simulink model "CAVE_MachE_Simulink_250904_Test"  (R2024a)
settings: configuration reference "ConfigSetDesktopFixedStep" (kept outside this file)
PreLoadFcn:
  | VSS_BICYCLE=Simulink.Variant('Dual=0');
  | VSS_DUAL=Simulink.Variant('Dual=1');
  | Dual=1;
  | load('DriveCycle2.mat')
PostLoadFcn:
  | if any(exist('dsrtsu_mdlpostloadfcn', 'file') ~= 0), dsrtsu_mdlpostloadfcn('Execute', bdroot); end
InitFcn:
  | , if any(exist('rtifpga_mdlclblib', 'file') ~= 0), rtifpga_mdlclblib('Init', bdroot); end,
  | , if any(exist('dsmpb_private', 'file') ~= 0), dsmpb_private('dsmpb_mdlclblib', 'Init', bdroot); end,
  | load('DriveCycle2.mat')
model workspace (MAT data in the model file):
  Gas = 0.383333333333
values from neighbouring files (symbols this model uses):
  CoastDown =     [Run_Simulink.mat]
  limitedMCT =     [Run_Simulink.mat]
  MCT =     [Run_Simulink.mat]
  pMCT =     [Run_Simulink.mat]
  RealSimPara =     [Run_Simulink.mat]
  Ref_speed = [13 13.007895099 13.015778396 13.023649891 13.031509584 13.039357475 13.047193564 13.055017851 13.062830336 13.070631019 13.0784199 13.086196979 ... (2669 elements, 2669x1)]    [Ref_speed_and_time.mat]
  Ref_time = [0 0.01 0.02 0.03 0.04 0.05 0.06 0.07 0.08 0.09 0.1 0.11 ... (2669 elements, 2669x1)]    [Ref_speed_and_time.mat]
  US06 =     [Run_Simulink.mat]
undefined symbols (not defined in the file or in its folder): AccelCmd, ActTqLF_Nm_, ActTqLR_Nm_, ActTqRF_Nm_, ActTqRR_Nm_, BattChargeLimitMaxPwr, BattChargeLimitSocBpts, BattChargeLimitTbl, BattChrgCapcty, BattDischargeLimitSocBpts, BattDischargeLimitTbl, BattDischargeMaxPwr, BattNumCellsParallel, BattNumCellsSeries, BattOpenVoltCapBpts, BattOpenVoltTbl, BattResistSocBpts, BattResistTbl, BattResistTempBpts, BrakeMaxPrs, BrakeMaxTrq, ChassisDistCg2FrontAxle, ChassisDistCg2RearAxle, ChassisVehMass, CltchCmd, DecelCmd, DiffRatio, DiscIntNeverNeededParam, EnvGravCnst, EnvPrs, EnvTemp, FuelSpecificGrav, GearCmd, h, InitStates, lgSw, MtrEffSpdBpts, MtrEffTbl, MtrEffTrqBpts, MtrPwrMax, MtrTrqMax, SteeringCmd, SupvsryCtrlRegenBrkCutOffTbl, SupvsryCtrlRegenSpdBpts, TestScnrioCycleNum, VEH
libraries: VSIGenLib x65, simulink x54, etargetslib x38, dsmpblib x24, vehdynlibtire x12, autolibshared x10, vehdynlibsuspension x7, vehdynlibtirecommon x7, autolibutils x5, CarMaker4SL x4, VsrLibWheel x4, autolibpowerinfoutils x3
(part 9 of 16)

== system CAVE_MachE_Simulink_250904_Test/Vehicle Under Test1/Vehicle/Vehicle Dynamics/Vehicle 7DOF/Longitudinal Wheels 4DOF/Tire2Veh ==
  Wheel : Inport
  Bus Selector7 : BusSelector  OutputSignals=Omega,Fx,Re,z,zdot,Kappa,Alpha
  Dead Zone2 : DeadZone  LowerValue=-5  UpperValue=5  ZeroCross=off
  Demux : Demux  Outputs=[2,2]
  Re : Terminator
  Unary Minus1 : UnaryMinus
  Unary Minus2 : UnaryMinus
  zdot : Terminator
  FwF : Outport  VectorParamsAs1DForOutWhenUnconnected=off
  FwR : Outport  Port=2  VectorParamsAs1DForOutWhenUnconnected=off
  z : Outport  Port=3  VectorParamsAs1DForOutWhenUnconnected=off
  Omega : Outport  Port=4  VectorParamsAs1DForOutWhenUnconnected=off
  Kappa : Outport  Port=5  VectorParamsAs1DForOutWhenUnconnected=off
  Alpha : Outport  Port=6  VectorParamsAs1DForOutWhenUnconnected=off
  wires:
  Bus Selector7/7 -> Alpha/1  "<Alpha>"
  Bus Selector7/3 -> Re/1  "<Re>"
  Unary Minus2/1 -> zdot/1  "zdot"
  Bus Selector7/6 -> Kappa/1  "<Kappa>"
  Demux/2 -> FwR/1
  Unary Minus1/1 -> z/1  "z"
  Bus Selector7/4 -> Unary Minus1/1  "<z>"
  Bus Selector7/5 -> Unary Minus2/1  "<zdot>"
  Bus Selector7/1 -> Omega/1  "<Omega>"
  Wheel/1 -> Bus Selector7/1
  Demux/1 -> FwF/1
  Dead Zone2/1 -> Demux/1  "Fx"
  Bus Selector7/2 -> Dead Zone2/1  "<Fx>"

== system CAVE_MachE_Simulink_250904_Test/Vehicle Under Test1/Vehicle/Vehicle Dynamics/Vehicle 7DOF/Longitudinal Wheels 4DOF/Tires ==
  AxlTrq : Inport
  BrkPrs : Inport  Port=2
  Vx : Inport  Port=3
  Vy : Inport  Port=4
  r : Inport  Port=5
  Camber : Inport  Port=6
  TirePrs : Inport  Port=7
  Fz : Inport  Port=8
  lam_mu : Inport  Port=9
  Gnd : Inport  Port=10
  4-by-1 Gnd : Subsystem
  4-by-1 Gnd1 : Subsystem
  4-by-1 Gnd2 : Subsystem
  4-by-1 Gnd3 : Subsystem
  Bus Creator : BusCreator  Inputs=12
  Subsystem : Subsystem
  Terminator1 : Terminator
  Terminator2 : Terminator
  Terminator3 : Terminator
  Wheel : Outport  VectorParamsAs1DForOutWhenUnconnected=off
  wires:
  Gnd/1 -> Subsystem/7(Gnd)
  lam_mu/1 -> Subsystem/6(lam_mu)
  Fz/1 -> Subsystem/5(Fz)
  TirePrs/1 -> Subsystem/4(TirePrs)
  Vx/1 -> Subsystem/3(Vx)
  BrkPrs/1 -> Subsystem/2(BrkPrs)
  AxlTrq/1 -> Subsystem/1(AxlTrq)
  4-by-1 Gnd3/1(Gnd) -> Bus Creator/12  "Alpha"
  Subsystem/8(Kappa) -> Bus Creator/11  "Kappa"
  4-by-1 Gnd2/1(Gnd) -> Bus Creator/7  "Mz"
  4-by-1 Gnd1/1(Gnd) -> Bus Creator/5  "Mx"
  4-by-1 Gnd/1(Gnd) -> Bus Creator/3  "Fy"
  Subsystem/4(My) -> Bus Creator/6  "My"
  Subsystem/3(FzOut) -> Bus Creator/4  "Fz"
  Subsystem/5(Re) -> Bus Creator/8  "Re"
  Subsystem/1(Omega) -> Bus Creator/1  "Omega"
  Subsystem/2(Fx) -> Bus Creator/2  "Fx"
  Subsystem/6(z) -> Bus Creator/9  "z"
  Subsystem/7(zdot) -> Bus Creator/10  "zdot"
  Bus Creator/1 -> Wheel/1
  r/1 -> Terminator3/1
  Camber/1 -> Terminator2/1
  Vy/1 -> Terminator1/1

== system CAVE_MachE_Simulink_250904_Test/Vehicle Under Test1/Vehicle/Vehicle Dynamics/Vehicle 7DOF/Longitudinal Wheels 4DOF/Veh2Tire ==
  AxlTrq : Inport
  BrkPrs : Inport  Port=2
  r : Inport  Port=3
  VehVel : Inport  Port=4
  WhlAng : Inport  Port=5
  Reshape3 : Reshape
  Reshape4 : Reshape
  Unary Minus : UnaryMinus
  Wheel to Body Transform : Subsystem
  T : Outport  VectorParamsAs1DForOutWhenUnconnected=off
  P : Outport  Port=2  VectorParamsAs1DForOutWhenUnconnected=off
  xdotAxle : Outport  Port=3  VectorParamsAs1DForOutWhenUnconnected=off
  ydotAxle : Outport  Port=4  VectorParamsAs1DForOutWhenUnconnected=off
  psidot : Outport  Port=5  VectorParamsAs1DForOutWhenUnconnected=off
  zdotAxle : Outport  Port=6  VectorParamsAs1DForOutWhenUnconnected=off
  wires:
  Reshape3/1 -> P/1
  Unary Minus/1 -> psidot/1
  Wheel to Body Transform/3(zdotWheel) -> zdotAxle/1  "Vz"
  WhlAng/1 -> Wheel to Body Transform/2(WhlAng)
  VehVel/1 -> Wheel to Body Transform/1(VelVeh)
  Reshape4/1 -> T/1
  r/1 -> Unary Minus/1
  Wheel to Body Transform/2(ydotWheel) -> ydotAxle/1  "Vy"
  Wheel to Body Transform/1(xdotWheel) -> xdotAxle/1  "Vx"
  AxlTrq/1 -> Reshape4/1
  BrkPrs/1 -> Reshape3/1

== system CAVE_MachE_Simulink_250904_Test/Vehicle Under Test1/Vehicle/Vehicle Dynamics/Vehicle 7DOF/Longitudinal Wheels 4DOF/Velocity and Vertical Load ==
  note: 1) Add Subsystem or Model blocks as valid variant choices.
      | 2) You cannot connect blocks at this level. At simulation, connectivity is automatically
      | determined, based on the active variant and port name matching.
  VehFdbk : Inport
  Bicycle : Subsystem  VariantControl=0
  Dual : Subsystem  VariantControl=1
  VehVel : Outport  VectorParamsAs1DForOutWhenUnconnected=off
  Fz : Outport  Port=2  PortDimensions=4  VectorParamsAs1DForOutWhenUnconnected=off

== system CAVE_MachE_Simulink_250904_Test/Vehicle Under Test1/Vehicle/Vehicle Dynamics/Vehicle 7DOF/Longitudinal Wheels 4DOF/Wheel Angles ==
  WheelAng : Inport
  Camber : Inport  Port=2
  Add1 : Sum
  Constant2 : Constant  Value=0
  Constant3 : Constant  Value=ones(1,4).*pi
  Demux : Demux  Outputs=2
  Demux1 : Demux
  Mux : Mux  Inputs=2
  Reshape : Reshape  OutputDimensionality=Row vector (2-D)
  Reshape1 : Reshape  OutputDimensionality=Row vector (2-D)
  Reshape2 : Reshape  OutputDimensionality=Row vector (2-D)
  Vector Concatenate3 : Concatenate  NumInputs=3  Mode=Multidimensional array
  Vector Concatenate4 : Concatenate  NumInputs=4
  WhlAngB : Outport  VectorParamsAs1DForOutWhenUnconnected=off
  wires:
  WheelAng/1 -> Demux1/1
  Camber/1 -> Reshape2/1
  Reshape2/1 -> Vector Concatenate3/2
  Reshape1/1 -> Vector Concatenate3/1
  Reshape/1 -> Vector Concatenate3/3
  Vector Concatenate3/1 -> WhlAngB/1
  Constant3/1 -> Reshape1/1
  Vector Concatenate4/1 -> Reshape/1
  Demux/2 -> Vector Concatenate4/4
  Demux/1 -> Vector Concatenate4/2
  Demux1/4 -> Mux/2
  Mux/1 -> Add1/1
  Demux1/1 -> Vector Concatenate4/1
  Demux1/3 -> Vector Concatenate4/3
  Add1/1 -> Demux/1
  Constant2/1 -> Add1/2
  Demux1/2 -> Mux/1

== system CAVE_MachE_Simulink_250904_Test/Vehicle Under Test1/Vehicle/Vehicle Dynamics/Vehicle 7DOF/Subsystem4/Subsystem ==
  CgXYZdot : Inport
  angles : Inport  Port=2
  Demux2 : Demux  Outputs=3
  Demux3 : Demux  Outputs=3
  Terminator{,1..4} (5 alike) : Terminator
  VehSpd : Outport
  wires:
  Demux2/1 -> VehSpd/1  "Xdot"
  angles/1 -> Demux3/1
  Demux2/3 -> Terminator1/1  "Zdot"
  Demux3/3 -> Terminator4/1  "psi"
  Demux3/1 -> Terminator2/1  "phi"
  Demux2/2 -> Terminator/1  "Ydot"
  Demux3/2 -> Terminator3/1  "theta"
  CgXYZdot/1 -> Demux2/1

== system CAVE_MachE_Simulink_250904_Test/Vehicle Under Test1/Vehicle/Vehicle Dynamics/Vehicle 7DOF/Vehicle Body 3DOF External Longitudinal Wheels/Bicycle ==
  WhlAng : Inport
  "FwF " : Inport  Port=2
  "FwR " : Inport  Port=3
  WindXYZ : Inport  Port=4
  Friction : Inport  Port=5
  Demux : Demux  Outputs=[2,2]
  Gain : Gain  Gain=.5
  Gain1 : Gain  Gain=.5
  Gain2 : Gain  Gain=.5
  Selector : Selector  InputPortWidth=4  IndexOptions=Index vector (dialog)  Indices=[1 2]  OutputSizes=1
  Signal Specification : SignalSpecification  Unit=1
  Signal Specification1 : SignalSpecification  Unit=rad
  Sum of Elements : Sum  Inputs=+
  Sum of Elements1 : Sum  Inputs=+
  Sum of Elements2 : Sum  Inputs=+
  Terminator{,1..5} (6 alike) : Terminator
  Vector Concatenate : Concatenate
  Vehicle Body 3DOF Single Track : autolibshared/Vehicle Body 3DOF Single Track  trackMode=Single (bicycle)  inputMode=External longitudinal forces  frontSteerMode=on  rearSteerMode=off  windMode=on  muMode=on  extFMode=off  extMMode=off  htchFMode=off  htchMMode=off  extXo=off  extpsio=off  extxdoto=off  extro=off  extYo=off  extTamb=off  extydoto=off  aMode=2  NF=ChassisNumFrontWhls  NR=ChassisNumRearWhls  m=ChassisVehMass  a=ChassisDistCg2FrontAxle  b=ChassisDistCg2RearAxle  h=ChassisCgHeight  dh=1  hh=0.2  X_o=0  xdot_o=20  CalphaMode=off  sigmaMode=on  d=0  hl=0  w=1.922.*[1 1]  Cy_f=15000  Cy_r=35000  sigma_f=.1  sigma_r=.1  alpha_f_brk=[-.1 .1]  Cy_f_data=[-9e3 9e3]  alpha_r_brk=[-.1 .1]  Cy_r_data=[-9e3 9e3]  Y_o=0  ydot_o=0  Izz=2500  psi_o=0  r_o=0  Af=ChassisFrontalArea  Cd=ChassisDragCoeff  Cl=.1  Cpm=.1  beta_w=[0:0.01:0.3]  Cs=[0:0.03:0.9]  Cym=[0:0.01:0.3]  Pabs=EnvPrs  Tair=EnvTemp  g=EnvGravCnst  mu=1  xdot_tol=1  Fznom=5000  Fxtire_sat=7e3*1e3  Fytire_sat=2e3*1e3  longOff=0  latOff=0  vertOff=.0112  wrapAng=off
  Wheel Positions : Subsystem
  " Info" : Outport  VectorParamsAs1DForOutWhenUnconnected=off
  XWheel : Outport  Port=2  Unit=m  VectorParamsAs1DForOutWhenUnconnected=off
  " YWheel" : Outport  Port=3  Unit=m  VectorParamsAs1DForOutWhenUnconnected=off
  wires:
  Vehicle Body 3DOF Single Track/3 -> Terminator5/1
  Vehicle Body 3DOF Single Track/2 -> Terminator4/1
  Vehicle Body 3DOF Single Track/5 -> Terminator3/1
  Vehicle Body 3DOF Single Track/4 -> Terminator2/1
  Wheel Positions/1(XWheel) -> XWheel/1
  Wheel Positions/2(YWheel) -> " YWheel"/1
  Signal Specification1/1 -> Vehicle Body 3DOF Single Track/1
  Signal Specification/1 -> ?
  Vector Concatenate/1 -> Signal Specification/1
  Gain2/1 -> Vector Concatenate/2
  Gain1/1 -> Vector Concatenate/1
  Demux/2 -> Sum of Elements2/1
  Sum of Elements2/1 -> Gain2/1
  Sum of Elements1/1 -> Gain1/1
  Friction/1 -> Demux/1
  Demux/1 -> Sum of Elements1/1
  Selector/1 -> Sum of Elements/1
  WindXYZ/1 -> ?
  Vehicle Body 3DOF Single Track/7 -> Terminator1/1
  Vehicle Body 3DOF Single Track/6 -> Terminator/1
  Sum of Elements/1 -> Gain/1
  Gain/1 -> Signal Specification1/1
  WhlAng/1 -> Selector/1
  Vehicle Body 3DOF Single Track/1 -> Wheel Positions/1(Info), " Info"/1
  "FwF "/1 -> Vehicle Body 3DOF Single Track/2
  "FwR "/1 -> Vehicle Body 3DOF Single Track/3

== system CAVE_MachE_Simulink_250904_Test/Vehicle Under Test1/Vehicle/Vehicle Dynamics/Vehicle 7DOF/Vehicle Body 3DOF External Longitudinal Wheels/Dual ==
  WhlAng : Inport
  "FwF " : Inport  Port=2
  "FwR " : Inport  Port=3
  WindXYZ : Inport  Port=4
  Friction : Inport  Port=5
  Reshape : Reshape  OutputDimensionality=Customize  OutputDimensions=[2,2]
  Selector : Selector  InputPortWidth=4  IndexOptions=Index vector (dialog)  Indices=[1 2]  OutputSizes=1
  Signal Specification : SignalSpecification  Unit=1
  Terminator{,1..5} (6 alike) : Terminator
  Vehicle Body 3DOF Dual Track : autolibshared/Vehicle Body 3DOF Single Track  trackMode=Dual  inputMode=External longitudinal forces  frontSteerMode=on  rearSteerMode=off  windMode=on  muMode=on  extFMode=off  extMMode=off  htchFMode=off  htchMMode=off  extXo=off  extpsio=off  extxdoto=off  extro=off  extYo=off  extTamb=off  extydoto=off  aMode=2  NF=ChassisNumFrontWhls  NR=ChassisNumRearWhls  m=ChassisVehMass  a=ChassisDistCg2FrontAxle  b=ChassisDistCg2RearAxle  h=ChassisCgHeight  dh=1  hh=0.2  X_o=0  xdot_o=InitStates(TestScnrioCycleNum).VehSpd  CalphaMode=off  sigmaMode=on  d=0  hl=0  w=1.9.*[1 1]  Cy_f=15000  Cy_r=35000  sigma_f=.1  sigma_r=.1  alpha_f_brk=[-.1 .1]  Cy_f_data=[-9e3 9e3]  alpha_r_brk=[-.1 .1]  Cy_r_data=[-9e3 9e3]  Y_o=0  ydot_o=0  Izz=2500  psi_o=0  r_o=0  Af=ChassisFrontalArea  Cd=ChassisDragCoeff  Cl=.1  Cpm=.1  beta_w=[0:0.01:0.3]  Cs=[0:0.03:0.9]  Cym=[0:0.01:0.3]  Pabs=EnvPrs  Tair=EnvTemp  g=EnvGravCnst  mu=1  xdot_tol=1  Fznom=5000  Fxtire_sat=7e3*1e3  Fytire_sat=2e3*1e3  longOff=0  latOff=0  vertOff=.0112  wrapAng=off
  Wheel Positions : Subsystem
  " Info" : Outport  VectorParamsAs1DForOutWhenUnconnected=off
  " XWheel" : Outport  Port=2  VectorParamsAs1DForOutWhenUnconnected=off
  " YWheel" : Outport  Port=3  VectorParamsAs1DForOutWhenUnconnected=off
  wires:
  "FwR "/1 -> Vehicle Body 3DOF Dual Track/3
  "FwF "/1 -> Vehicle Body 3DOF Dual Track/2
  WindXYZ/1 -> ?
  Signal Specification/1 -> ?
  Vehicle Body 3DOF Dual Track/7 -> Terminator/1
  Vehicle Body 3DOF Dual Track/5 -> Terminator3/1
  Vehicle Body 3DOF Dual Track/4 -> Terminator2/1
  Vehicle Body 3DOF Dual Track/6 -> Terminator1/1
  Vehicle Body 3DOF Dual Track/3 -> Terminator5/1
  Vehicle Body 3DOF Dual Track/2 -> Terminator4/1
  Wheel Positions/2(YWheel) -> " YWheel"/1
  Wheel Positions/1(XWheel) -> " XWheel"/1
  Vehicle Body 3DOF Dual Track/1 -> Wheel Positions/1(Info), " Info"/1
  Reshape/1 -> Signal Specification/1
  Friction/1 -> Reshape/1
  Selector/1 -> Vehicle Body 3DOF Dual Track/1
  WhlAng/1 -> Selector/1

== system CAVE_MachE_Simulink_250904_Test/Vehicle Under Test1/Vehicle/Vehicle Dynamics/Vehicle Longitudinal/Longitudinal Wheels/Front Diff Wheels ==
  BrkPrs : Inport
  AxleTorq : Inport  Port=2
  Add2 : Sum
  Bus Creator : BusCreator  Inputs=3
  Bus Creator5 : BusCreator  Inputs=1
  Bus Selector6 : BusSelector  OutputSignals=VehSpd,FrcZ
  Bus Selector7 : BusSelector  OutputSignals=VehSpd,FrcZ
  Selector : Selector  InputPortWidth=4  IndexOptions=Index vector (dialog)  Indices=1  OutputSizes=1
  Selector1 : Selector  InputPortWidth=4  IndexOptions=Index vector (dialog)  Indices=2  OutputSizes=1
  Selector2 : Selector  InputPortWidth=4  IndexOptions=Index vector (dialog)  Indices=1  OutputSizes=1
  Selector3 : Selector  InputPortWidth=4  IndexOptions=Index vector (dialog)  Indices=2  OutputSizes=1
  Simple Longitudinal Wheel 1 : VsrLibWheel/Simple Longitudinal Wheel  TireLoadedRadius=WhlRearLoadedRadius  C_rr=WhlRollingResistCnst  MaxBrkTrq=BrakeMaxTrq  MaxBrkPrs=BrakeMaxPrs  w_thresh=WhlSimVelTol
  Simple Longitudinal Wheel 2 : VsrLibWheel/Simple Longitudinal Wheel  TireLoadedRadius=WhlRearLoadedRadius  C_rr=WhlRollingResistCnst  MaxBrkTrq=BrakeMaxTrq  MaxBrkPrs=BrakeMaxPrs  w_thresh=WhlSimVelTol
  Terminator3 : Terminator
  Two-Way Connection6 : TwoWayConnection
  DiffAxle : PMIOPort  Side=Right
  Info : Outport
  wires:
  Simple Longitudinal Wheel 2/3 -> Bus Creator/3  "Omega2"
  Simple Longitudinal Wheel 1/1 -> Bus Creator/1  "WhlFrontInfo"
  Bus Creator/1 -> Info/1
  Simple Longitudinal Wheel 1/3 -> Bus Creator/2  "Omega1"
  Selector3/1 -> Simple Longitudinal Wheel 2/1
  Selector1/1 -> Simple Longitudinal Wheel 2/2
  Selector/1 -> Simple Longitudinal Wheel 1/2
  AxleTorq/1 -> Selector/1, Selector1/1
  Selector2/1 -> Simple Longitudinal Wheel 1/1
  Simple Longitudinal Wheel 2/1 -> Terminator3/1
  Bus Creator5/1 -> Two-Way Connection6/1
  Simple Longitudinal Wheel 2/2 -> Add2/2  "Spd"
  Add2/1 -> Bus Creator5/1  "FrcX"
  Two-Way Connection6/1 -> Bus Selector6/1, Bus Selector7/1
  Bus Selector7/2 -> Simple Longitudinal Wheel 2/4  "<FrcZ>"
  Bus Selector6/1 -> Simple Longitudinal Wheel 1/3  "<VehSpd>"
  Bus Selector7/1 -> Simple Longitudinal Wheel 2/3  "<VehSpd>"
  Simple Longitudinal Wheel 1/2 -> Add2/1
  BrkPrs/1 -> Selector2/1, Selector3/1
  Bus Selector6/2 -> Simple Longitudinal Wheel 1/4  "<FrcZ>"
  connections:
  DiffAxle/RConn1 -- Two-Way Connection6/RConn1

== system CAVE_MachE_Simulink_250904_Test/Vehicle Under Test1/Vehicle/Vehicle Dynamics/Vehicle Longitudinal/Longitudinal Wheels/Rear Wheels ==
  BrkPrs : Inport
  Add2 : Sum
  Bus Creator : BusCreator  Inputs=3
  Bus Creator5 : BusCreator  Inputs=1
  Bus Selector6 : BusSelector  OutputSignals=VehSpd,FrcZ
  Bus Selector7 : BusSelector  OutputSignals=VehSpd,FrcZ
  Ground : Ground
  Selector : Selector  InputPortWidth=4  IndexOptions=Index vector (dialog)  Indices=3  OutputSizes=1
  Selector1 : Selector  InputPortWidth=4  IndexOptions=Index vector (dialog)  Indices=4  OutputSizes=1
  Simple Longitudinal Wheel : VsrLibWheel/Simple Longitudinal Wheel  TireLoadedRadius=WhlFrontLoadedRadius  C_rr=WhlRollingResistCnst  MaxBrkTrq=BrakeMaxTrq  MaxBrkPrs=BrakeMaxPrs  w_thresh=WhlSimVelTol
  Simple Longitudinal Wheel1 : VsrLibWheel/Simple Longitudinal Wheel  TireLoadedRadius=WhlFrontLoadedRadius  C_rr=WhlRollingResistCnst  MaxBrkTrq=BrakeMaxTrq  MaxBrkPrs=BrakeMaxPrs  w_thresh=WhlSimVelTol
  Terminator3 : Terminator
  Two-Way Connection6 : TwoWayConnection
  DiffAxle : PMIOPort  Side=Right
  Info : Outport
  wires:
  Bus Creator/1 -> Info/1
  Simple Longitudinal Wheel/1 -> Bus Creator/1  "WhlRearInfo"
  Selector1/1 -> Simple Longitudinal Wheel1/1
  Selector/1 -> Simple Longitudinal Wheel/1
  Bus Selector6/2 -> Simple Longitudinal Wheel/4  "<FrcZ>"
  BrkPrs/1 -> Selector/1, Selector1/1
  Simple Longitudinal Wheel/2 -> Add2/1
  Bus Selector7/1 -> Simple Longitudinal Wheel1/3  "<VehSpd>"
  Bus Selector6/1 -> Simple Longitudinal Wheel/3  "<VehSpd>"
  Bus Selector7/2 -> Simple Longitudinal Wheel1/4  "<FrcZ>"
  Two-Way Connection6/1 -> Bus Selector6/1, Bus Selector7/1
  Add2/1 -> Bus Creator5/1  "FrcX"
  Simple Longitudinal Wheel1/2 -> Add2/2  "Spd"
  Bus Creator5/1 -> Two-Way Connection6/1
  Simple Longitudinal Wheel/3 -> Bus Creator/2  "Omega3"
  Ground/1 -> Simple Longitudinal Wheel1/2, Simple Longitudinal Wheel/2
  Simple Longitudinal Wheel1/3 -> Bus Creator/3  "Omega4"
  Simple Longitudinal Wheel1/1 -> Terminator3/1
  connections:
  DiffAxle/RConn1 -- Two-Way Connection6/RConn1

== system CAVE_MachE_Simulink_250904_Test/Vehicle Under Test1/Vehicle/Vehicle Dynamics/Vehicle Longitudinal/Vehicle Body/Logitudinal Vehicle Body ==
  RoadGrade : Inport
  WindVel : Inport  Port=2  Unit=m/s
  Bus Creator : BusCreator  Inputs=2
  Bus Creator1 : BusCreator  Inputs=2
  Bus Selector : BusSelector  OutputSignals=FrcX
  Bus Selector1 : BusSelector  OutputSignals=BdyFrm.Cg.Vel.xdot,BdyFrm.Cg.Disp.x
  Bus Selector3 : BusSelector  OutputSignals=FrcX
  Signal Specification3 : SignalSpecification  Unit=N
  Signal Specification4 : SignalSpecification  Unit=N
  Transfer Fcn : TransferFcn  Denominator=[0.01 1]
  Transfer Fcn1 : TransferFcn  Denominator=[0.01 1]
  Two-Way Connection2 : TwoWayConnection
  Two-Way Connection8 : TwoWayConnection
  Unit Conversion : UnitConversion
  Vehicle Body 1DOF Longitudinal : autolibshared/Vehicle Body 1DOF Longitudinal  VariantControl=SL  extFMode=off  extMMode=off  extTamb=off  wind3D=off  aMode=1  NF=ChassisNumFrontWhls  NR=ChassisNumRearWhls  m=ChassisVehMass  a=ChassisDistCg2FrontAxle  b=ChassisDistCg2RearAxle  h=ChassisCgHeight  Cd=ChassisDragCoeff  Cl=0  Cpm=0  Af=ChassisFrontalArea  x_o=0  xdot_o=InitStates(TestScnrioCycleNum).VehSpd  Pabs=EnvPrs  T=EnvTemp  g=EnvGravCnst
      settings: LibrarySourceBlock=autolibvehdynlong/Vehicle Body 1DOF Longitudinal
  Front : PMIOPort  Side=Left
  Rear : PMIOPort  Port=2  Side=Left
  VehSpd : Outport  VectorParamsAs1DForOutWhenUnconnected=off
  VehDist : Outport  Port=2  VectorParamsAs1DForOutWhenUnconnected=off
  FrontAxleFrc : Outport  Port=3  VectorParamsAs1DForOutWhenUnconnected=off
  RearAxleFrc : Outport  Port=4  VectorParamsAs1DForOutWhenUnconnected=off
  wires:
  Bus Selector3/1 -> Transfer Fcn/1  "<FrcX>"
  Bus Creator1/1 -> Two-Way Connection2/1
  Transfer Fcn1/1 -> Signal Specification4/1
  Transfer Fcn/1 -> Signal Specification3/1
  Signal Specification4/1 -> Vehicle Body 1DOF Longitudinal/1, FrontAxleFrc/1  "FrontAxleFrc"
  Unit Conversion/1 -> Vehicle Body 1DOF Longitudinal/3
  Bus Selector1/2 -> VehDist/1  "<x>"
  Bus Selector1/1 -> VehSpd/1  "<xdot>"
  Vehicle Body 1DOF Longitudinal/4 -> Bus Creator1/2  "FrcZ"
  Two-Way Connection2/1 -> Bus Selector3/1
  WindVel/1 -> Vehicle Body 1DOF Longitudinal/4
  Vehicle Body 1DOF Longitudinal/3 -> Bus Creator/2  "FrcZ"
  Bus Creator/1 -> Two-Way Connection8/1
  Signal Specification3/1 -> Vehicle Body 1DOF Longitudinal/2, RearAxleFrc/1  "RearAxleFrc"
  Vehicle Body 1DOF Longitudinal/1 -> Bus Selector1/1  "Veh"
  Vehicle Body 1DOF Longitudinal/2 -> Bus Creator1/1, Bus Creator/1  "VehSpd"
  Bus Selector/1 -> Transfer Fcn1/1  "<FrcX>"
  RoadGrade/1 -> Unit Conversion/1
  Two-Way Connection8/1 -> Bus Selector/1
  connections:
  Two-Way Connection2/RConn1 -- Rear/RConn1
  Two-Way Connection8/RConn1 -- Front/RConn1

== system CAVE_MachE_Simulink_250904_Test/Vehicle Under Test1/Vehicle/Vehicle Dynamics/Vehicle Longitudinal/Vehicle Body/Subsystem1 ==
  VehSpd : Inport
  VehDist : Inport  Port=2
  FrontAxleFrc : Inport  Port=3
  RearAxleFrc : Inport  Port=4
  Bus Creator : BusCreator  Inputs=4
  ChassisPlant : Outport
  wires:
  RearAxleFrc/1 -> Bus Creator/4  "RearAxleFrc"
  FrontAxleFrc/1 -> Bus Creator/3  "FrontAxleFrc"
  Bus Creator/1 -> ChassisPlant/1  "ChassisPlant"
  VehDist/1 -> Bus Creator/2  "VehDist"
  VehSpd/1 -> Bus Creator/1  "VehSpd"

== system CAVE_MachE_Simulink_250904_Test/Vehicle Under Test1/Vehicle/Actuation and Outputs/MOOG Brake Actuator/ CAN Settings/ CAN diagnostic Counter/Timer ==
  Reset : Inport
  Constant : Constant
  Integrator : Integrator  ExternalReset=level  LimitOutput=on  LowerSaturationLimit=0  ZeroCross=off
  Timer : Outport
  wires:
  Constant/1 -> Integrator/1
  Reset/1 -> Integrator/2
  Integrator/1 -> Timer/1

== system CAVE_MachE_Simulink_250904_Test/Vehicle Under Test1/Vehicle/Battery/Battery/Lithium Ion Battery Pack1/Datasheet Battery Internal/Datasheet Battery ==
  CapInit : Inport  Unit=A*hr
  BattCurr : Inport  Port=2  Unit=A
  BattTemp : Inport  Port=3  Unit=K
  Charge Model : Subsystem
  State of Charge Capacity : Subsystem
  Voltage and Power Calculation : Subsystem
  LdCurrFeed : Outport  Unit=A  VectorParamsAs1DForOutWhenUnconnected=off
  OutVoltUnfilt : Outport  Port=2  Unit=V  VectorParamsAs1DForOutWhenUnconnected=off
  LdAmpHr : Outport  Port=3  Unit=A*hr  VectorParamsAs1DForOutWhenUnconnected=off
  BattSoc : Outport  Port=4  Unit=1  VectorParamsAs1DForOutWhenUnconnected=off
  BattPwrLoss : Outport  Port=5  Unit=V  VectorParamsAs1DForOutWhenUnconnected=off
  wires:
  BattCurr/1 -> LdCurrFeed/1, Voltage and Power Calculation/2(LdAmp), Charge Model/1(LdAmp)
  Voltage and Power Calculation/1(OutVolt) -> OutVoltUnfilt/1
  Charge Model/1(LdAmpHr) -> State of Charge Capacity/1(LdAmpHr), LdAmpHr/1
  State of Charge Capacity/1(CapSOC) -> Voltage and Power Calculation/1(CapSOC), BattSoc/1
  BattTemp/1 -> Voltage and Power Calculation/3(BattTemp)
  CapInit/1 -> Charge Model/2(CapInit)
  Voltage and Power Calculation/2(BattPwrLoss) -> BattPwrLoss/1

== system CAVE_MachE_Simulink_250904_Test/Vehicle Under Test1/Vehicle/Driver and Drive Cycle/Driver and PI with FF Control/Speed controller set/In-house CAVE/In-house Speed Controller ==
  note: ToDo: Maybe do something clever with FF and Brake, or maybe not.
      | Bleed FF based on refspd derivative
  RefSpd : Inport
  VehicleSpeed : Inport  Port=2
  Add : Sum  Inputs=+-
  Compare To Constant1 : simulink/Logic and Bit Operations/Compare To Constant  relop=<=  const=0.1  OutDataTypeStr=boolean  ZeroCross=off
  Compare To Constant3 : simulink/Logic and Bit Operations/Compare To Constant  relop=<=  const=0  OutDataTypeStr=boolean  ZeroCross=off
  Constant : Constant  Value=0
  Detect Fall Negative : simulink/Logic and Bit Operations/Detect Fall Negative  vinit=0  OutDataTypeStr=boolean
  Detect Rise Positive : simulink/Logic and Bit Operations/Detect Rise Positive  vinit=0  OutDataTypeStr=boolean
  Feedforward : Lookup_n-D  NumberOfTableDimensions=1  BreakpointsForDimension1="[0 10    20    30    40    50    60    70    80    90   100   110   120   130   140   150   160]"  Table="[0\t3.5\t12.5\t16\t20\t21\t22\t24.5\t26\t29.5\t32\t33\t34\t36\t37\t38\t39]"  ExtrapMethod=Clip  InternalRulePriority=Speed  RndMeth=Simplest
  Feedforward1 : Lookup_n-D  NumberOfTableDimensions=1  BreakpointsForDimension1="[0 10    20    30    40    50    60    70    80    90   100   110   120   130   140   150   160]"  Table="[0 2.6021    4.7790    6.8575    8.1555    9.4176   10.7914   12.3245   14.1570   15.9699   17.4605   19.0355   21.3079   22.8407   25.3373   26.9453   28.6975]"  ExtrapMethod=Clip  InternalRulePriority=Speed  RndMeth=Simplest
  FeedforwardGain : Gain
  Gain : Gain  Gain=-1
  Ground1 : Ground
  Ki : Gain
  Kp : Gain  Gain=10
  Limits [-50,50] : Integrator  ExternalReset=either  LimitOutput=on  UpperSaturationLimit=50  LowerSaturationLimit=-50
  Logical Operator : Logic  Operator=OR  Inputs=3  AllPortsSameDT=off  OutDataTypeStr=boolean
  Lowpass Filter : TransferFcn  Denominator=[.02 1]
  Memory : Memory
  Memory1 : Memory
  Min threshold for Brake switch : Constant  Value=0
  Product1 : Product  RndMeth=Zero
  Proportional Gain Scheduling : Lookup_n-D  NumberOfTableDimensions=1  BreakpointsForDimension1=[ 0 30 70]  IndexSearchMethod=Linear search  BeginIndexSearchUsingPreviousIndexResult=on  Table=[1 1 1]  ExtrapMethod=Clip  UseLastTableValue=on  RndMeth=Simplest
  Relational Operator : RelationalOperator  Operator=>  OutDataTypeStr=boolean  InputSameDT=off
  Sum : Sum  Inputs=|+-
  Sum1 : Sum  Inputs=+++
  Switch{1..4} (4 alike) : Switch  Criteria=u2 > Threshold  SaturateOnIntegerOverflow=off  InputSameDT=off
  standstill brake [0,100] : Constant  Value=50
  AcceleratorPedalPos : Outport  VectorParamsAs1DForOutWhenUnconnected=off
  BrakePedalPos : Outport  Port=2  VectorParamsAs1DForOutWhenUnconnected=off
  BrakeSwitch : Outport  Port=3  VectorParamsAs1DForOutWhenUnconnected=off
  wires:
  FeedforwardGain/1 -> Sum1/3  "Driver_FdfwdTerm_pct"
  Feedforward1/1 -> FeedforwardGain/1
  Product1/1 -> Sum1/2  "Driver_PropTerm_pct"
  Proportional Gain Scheduling/1 -> Product1/2
  Switch4/1 -> BrakePedalPos/1  "BrakePedalPos_pct"
  standstill brake [0,100]/1 -> Switch4/1
  Constant/1 -> Switch3/1
  Switch3/1 -> AcceleratorPedalPos/1  "AcceleratorPedalPos_pct"
  Compare To Constant1/1 -> Switch4/2, Switch3/2
  Memory1/1 -> Add/1
  Memory/1 -> Add/2
  Add/1 -> Detect Rise Positive/1, Detect Fall Negative/1
  Detect Fall Negative/1 -> Logical Operator/3
  Detect Rise Positive/1 -> Logical Operator/2
  Compare To Constant3/1 -> Logical Operator/1
  Logical Operator/1 -> Limits [-50,50]/2
  Gain/1 -> Switch2/2, Switch2/1
  Ground1/1 -> Switch1/3, Switch2/3
  Ki/1 -> Limits [-50,50]/1
  Sum1/1 -> Switch1/2, Switch1/1, Gain/1  "Driver_TotCmdPreLim_pct"
  Relational Operator/1 -> BrakeSwitch/1  "BrakeSwitch"
  Lowpass Filter/1 -> Sum/2  "VS_Flt"
  Switch2/1 -> Memory/1, Relational Operator/1, Switch4/3  "BrakePedalPosPre_pct"
  VehicleSpeed/1 -> Lowpass Filter/1, Proportional Gain Scheduling/1
  Limits [-50,50]/1 -> Sum1/1  "Driver_IntTerm_pct"
  Sum/1 -> Ki/1, Kp/1  "SpdErr"
  RefSpd/1 -> Sum/1, Compare To Constant3/1, Compare To Constant1/1, Feedforward1/1  "RefSpd"
  Switch1/1 -> Memory1/1, Switch3/3  "AcceleratorPedalPosPre_pct"
  Min threshold for Brake switch/1 -> Relational Operator/2
  Kp/1 -> Product1/1

== system CAVE_MachE_Simulink_250904_Test/Vehicle Under Test1/Vehicle/Driver and Drive Cycle/Driver and PI with FF Control/Speed controller set/Predictive/Longitudinal Driver1 ==
  note: To switch variants, right-click on this subsystem (from one level above) and chose:
      | Variant, Active choice, <your selection>
  "Vref " : Inport
  "Vfdbk " : Inport  Port=2
  Longitudinal Driver : Subsystem  VariantControl=0
      mask Display: image('LongitudinalDriver.png', 'center')
  Open Loop : Subsystem  VariantControl=1
      mask Display: disp('Open Loop')
  " OpCmds" : Outport  VectorParamsAs1DForOutWhenUnconnected=off

== system CAVE_MachE_Simulink_250904_Test/Vehicle Under Test1/Vehicle/Driver and Drive Cycle/Driver and PI with FF Control/Speed controller set/Speed tracking controller/In-house CAVE ==
  note: BrakeSwitch
  RefSpd [km/hr] : Inport
  In2 : Inport  Port=2
  Vehicle Speed Controller : Subsystem
  AccelPedalCmd : Outport
  BrakePedalCmd : Outport  Port=2
  Out3 : Outport  Port=3
  wires:
  Vehicle Speed Controller/1(AcceleratorPedalPos) -> AccelPedalCmd/1  "AccelPedalCmd"
  In2/1 -> Vehicle Speed Controller/2(VehicleSpeed)
  RefSpd [km/hr]/1 -> Vehicle Speed Controller/1(RefSpd)
  Vehicle Speed Controller/2(BrakePedalPos) -> BrakePedalCmd/1  "BrakePedalCmd"
  Vehicle Speed Controller/3(BrakeSwitch) -> Out3/1

== system CAVE_MachE_Simulink_250904_Test/Vehicle Under Test1/Vehicle/Driver and Drive Cycle/Driver and PI with FF Control/Speed controller set/Speed tracking controller/PIF ==
  RefSpd [km/hr] : Inport
  In2 : Inport  Port=2
  Compare To Constant1 : simulink/Logic and Bit Operations/Compare To Constant  relop=<=  const=0.1  OutDataTypeStr=boolean  ZeroCross=off
  Constant : Constant  Value=0
  Constant1 : Constant  Value=0
  Gain : Gain  Gain=1/3.6
  Gain1 : Gain  Gain=1/3.6
  Gain2 : Gain  Gain=100
  Gain3 : Gain  Gain=100
  Longitudinal Driver : autolibshared/Longitudinal Driver  extAccelOvr=off  extDecelOvr=off  extAccelHld=off  extDecelHld=off  extAccelZero=off  extDecelZero=off  cntrlType=PI  shftType=None  velUnits=m/s  gearOut=off  Kp=2  Ki=2  Kff=.1*0.4  Kg=0  VehVelVec=[0 100]  KffVec=[.1 .1]  KpVec=[10 10]  KiVec=[5 5]  KgVec=[0 0]  m=1500  Kpt=3000  tau=.1  L=2  aR=200  bR=2.5  cR=.5  g=9.81  vnom=1  Kaw=1  tauerr=.01  tauPt=2  GearInit=0  tShift=.1  pdlVec=[0.1 0.4 0.5 0.9]  upShftTbl=[-1 12.9375 26.4375 39.9375 51.18749999999999 62.4375 72.84375 83.25;-1 16.3125 29.8125 43.3125 54.5624 65.8125 76.78125 87.75;-1 19.6875 33.1875 46.68749999999999 57.9375 69.1875 80.71875 92.25;-1 33 52.5 77.25 100.5 138.75 161.875 185]  dwnShftTbl=[1 9.5625 23.0625 36.5625 47.8125 59.0625 68.90625 78.75;1 12.9375 26.4375 39.9375 51.18749999999999 62.4375 72.84375 83.25;1 16.3125 29.8125 43.3125 54.562499 65.8125 76.78125 87.75;1 19.6875 33.1875 46.68749999999999 57.9375 69.1875 80.71875 92.25]  tClutch=.5  tRev=.5  tPark=120  aMode=2  UpGearVec="[0  1  2  3  4  5  6  7]"  DownGearVec="[1  2  3  4  5  6  7  8]"
      settings: LibrarySourceBlock=vehdynlibdriver/Longitudinal Driver
  Lowpass Filter : TransferFcn  Denominator=[.01 1]
  Min threshold for Brake switch : Constant  Value=0
  Relational Operator : RelationalOperator  Operator=>  OutDataTypeStr=boolean  InputSameDT=off
  Switch3 : Switch  Criteria=u2 > Threshold  SaturateOnIntegerOverflow=off  InputSameDT=off
  Switch4 : Switch  Criteria=u2 > Threshold  SaturateOnIntegerOverflow=off  InputSameDT=off
  Terminator : Terminator
  standstill brake [0,1] : Constant  Value=0.5
  AccelPedalCmd : Outport
  BrakePedalCmd : Outport  Port=2
  Out3 : Outport  Port=3
  wires:
  Lowpass Filter/1 -> Gain1/1  "VS_Flt"
  Switch4/1 -> Gain3/1  "BrakePedalPos_pct"
  Switch3/1 -> Gain2/1  "AcceleratorPedalPos_pct"
  standstill brake [0,1]/1 -> Switch4/1
  Compare To Constant1/1 -> Switch3/2, Switch4/2
  Constant/1 -> Switch3/1
  Longitudinal Driver/2 -> Switch3/3  "AcceleratorPedalPosPre_pct"
  Longitudinal Driver/1 -> Terminator/1
  Gain2/1 -> AccelPedalCmd/1  "AccelPedalCmd"
  Gain3/1 -> BrakePedalCmd/1  "BrakePedalCmd"
  In2/1 -> Lowpass Filter/1
  RefSpd [km/hr]/1 -> Gain/1
  Constant1/1 -> Longitudinal Driver/3
  Gain/1 -> Longitudinal Driver/1, Compare To Constant1/1
  Longitudinal Driver/3 -> Relational Operator/1, Switch4/3  "BrakePedalPosPre_pct"
  Relational Operator/1 -> Out3/1  "BrakeSwitch"
  Min threshold for Brake switch/1 -> Relational Operator/2
  Gain1/1 -> Longitudinal Driver/2

== system CAVE_MachE_Simulink_250904_Test/Vehicle Under Test1/Vehicle/Driver and Drive Cycle/Driver and PI with FF Control/Speed controller set/Speed tracking controller/Predictive ==
  RefSpd [km/hr] : Inport
  In2 : Inport  Port=2
  Compare To Constant1 : simulink/Logic and Bit Operations/Compare To Constant  relop=<=  const=0.1  OutDataTypeStr=boolean  ZeroCross=off
  Constant : Constant  Value=0
  Constant1 : Constant  Value=0
  Gain : Gain  Gain=1/3.6
  Gain1 : Gain  Gain=1/3.6
  Gain4 : Gain  Gain=100
  Gain5 : Gain  Gain=100
  Longitudinal Driver : autolibshared/Longitudinal Driver  extAccelOvr=off  extDecelOvr=off  extAccelHld=off  extDecelHld=off  extAccelZero=off  extDecelZero=off  cntrlType=Predictive  shftType=None  velUnits=m/s  gearOut=off  Kp=10  Ki=5  Kff=.1  Kg=0  VehVelVec=[0 100]  KffVec=[.1 .1]  KpVec=[10 10]  KiVec=[5 5]  KgVec=[0 0]  m=2040  Kpt=6200  tau=0.1  L=3  aR=200/10  bR=2.5/10  cR=.3  g=9.807  vnom=5  Kaw=1  tauerr=.01  tauPt=2  GearInit=0  tShift=.1  pdlVec=[0.1 0.4 0.5 0.9]  upShftTbl=[-1 12.9375 26.4375 39.9375 51.18749999999999 62.4375 72.84375 83.25;-1 16.3125 29.8125 43.3125 54.5624 65.8125 76.78125 87.75;-1 19.6875 33.1875 46.68749999999999 57.9375 69.1875 80.71875 92.25;-1 33 52.5 77.25 100.5 138.75 161.875 185]  dwnShftTbl=[1 9.5625 23.0625 36.5625 47.8125 59.0625 68.90625 78.75;1 12.9375 26.4375 39.9375 51.18749999999999 62.4375 72.84375 83.25;1 16.3125 29.8125 43.3125 54.562499 65.8125 76.78125 87.75;1 19.6875 33.1875 46.68749999999999 57.9375 69.1875 80.71875 92.25]  tClutch=.5  tRev=.5  tPark=120  aMode=2  UpGearVec="[0  1  2  3  4  5  6  7]"  DownGearVec="[1  2  3  4  5  6  7  8]"
      settings: LibrarySourceBlock=vehdynlibdriver/Longitudinal Driver
  Lowpass Filter : TransferFcn  Denominator=[.02 1]
  Min threshold for Brake switch : Constant  Value=0
  Relational Operator : RelationalOperator  Operator=>  OutDataTypeStr=boolean  InputSameDT=off
  Switch3 : Switch  Criteria=u2 > Threshold  SaturateOnIntegerOverflow=off  InputSameDT=off
  Switch4 : Switch  Criteria=u2 > Threshold  SaturateOnIntegerOverflow=off  InputSameDT=off
  Terminator : Terminator
  standstill brake [0,1] : Constant  Value=0.5
  AccelPedalCmd : Outport
  BrakePedalCmd : Outport  Port=2
  Out3 : Outport  Port=3
  wires:
  Lowpass Filter/1 -> Gain1/1  "VS_Flt"
  Longitudinal Driver/2 -> Switch3/3  "AcceleratorPedalPosPre_pct"
  Gain5/1 -> BrakePedalCmd/1  "BrakePedalCmd"
  Gain/1 -> Longitudinal Driver/1, Compare To Constant1/1
  Gain4/1 -> AccelPedalCmd/1  "AccelPedalCmd"
  Constant/1 -> Switch3/1
  Compare To Constant1/1 -> Switch3/2, Switch4/2
  Switch3/1 -> Gain4/1  "AcceleratorPedalPos_pct"
  Switch4/1 -> Gain5/1  "BrakePedalPos_pct"
  Longitudinal Driver/3 -> Relational Operator/1, Switch4/3  "BrakePedalPosPre_pct"
  standstill brake [0,1]/1 -> Switch4/1
  Longitudinal Driver/1 -> Terminator/1
  In2/1 -> Lowpass Filter/1
  RefSpd [km/hr]/1 -> Gain/1
  Constant1/1 -> Longitudinal Driver/3
  Relational Operator/1 -> Out3/1  "BrakeSwitch"
  Min threshold for Brake switch/1 -> Relational Operator/2
  Gain1/1 -> Longitudinal Driver/2

== system CAVE_MachE_Simulink_250904_Test/Vehicle Under Test1/Vehicle/Powertrain Supervisory Controller /Engine Torque Command/Motor Torque Arbitration and Power Management/Power Management/Check Within Limits ==
  up : Inport
  u : Inport  Port=2
  lo : Inport  Port=3
  Compare To Zero : simulink/Logic and Bit Operations/Compare To Zero  relop=>=  OutDataTypeStr=boolean
  Compare To Zero1 : simulink/Logic and Bit Operations/Compare To Zero  relop=<=  OutDataTypeStr=boolean
  Logical Operator : Logic  AllPortsSameDT=off  OutDataTypeStr=boolean
  Saturation Dynamic1 : simulink/Discontinuities/Saturation Dynamic  OutMin=[]  OutMax=[]  OutDataTypeStr=Inherit: Same as second input  OutDataType=fixdt(1, 16)  OutScaling=2^-10  DoSatur=off
  Subtract : Sum  Inputs=+-
  Subtract1 : Sum  Inputs=-+
  InLimit : Outport  VectorParamsAs1DForOutWhenUnconnected=off
  y : Outport  Port=2  VectorParamsAs1DForOutWhenUnconnected=off
  wires:
  Saturation Dynamic1/1 -> y/1
  lo/1 -> Subtract1/2, Saturation Dynamic1/3
  up/1 -> Subtract/1, Saturation Dynamic1/1
  u/1 -> Subtract1/1, Subtract/2, Saturation Dynamic1/2
  Subtract/1 -> Compare To Zero/1
  Subtract1/1 -> Compare To Zero1/1
  Compare To Zero/1 -> Logical Operator/1
  Compare To Zero1/1 -> Logical Operator/2
  Logical Operator/1 -> InLimit/1

== system CAVE_MachE_Simulink_250904_Test/Vehicle Under Test1/Vehicle/Powertrain Supervisory Controller /Engine Torque Command/Motor Torque Arbitration and Power Management/Power Management/Mech to Elec Power Estimate ==
  note: Check if Motoring
      | or Generating
  note: Using an Efficiency Map, we can estimate the
      | Electric Power from the Mechanical  Torque Request.
  note: Pelec_req = Pmech_req*Eff^k,
      | k = -1 if Motoring >= 0,
      | k = 1 if Generating < 0
  MotTrqCmd : Inport
  MotSpd : Inport  Port=2
  Abs : Abs  SaturateOnIntegerOverflow=off
  Abs1 : Abs  SaturateOnIntegerOverflow=off
  Constant1 : Constant  Value=-1  SampleTime=-1
  Constant2 : Constant  SampleTime=-1
  Eff Map : Lookup_n-D  BreakpointsForDimension1=MtrEffSpdBpts  BreakpointsForDimension2=MtrEffTrqBpts  Table=MtrEffTbl  ExtrapMethod=Clip  UseLastTableValue=on  InternalRulePriority=Speed  OutDataTypeStr=Inherit: Inherit from 'Table data'  RndMeth=Simplest
      settings: InputPortMap=u0,u1
  Gain1 : Gain  Gain=1/100
  Math Function : Math  Operator=pow  SignedPower=on  OutputSignalType=real
  Product : Product
  Product3 : Product
  Product4 : Product
  Switch2 : Switch  SaturateOnIntegerOverflow=off  InputSameDT=off
  rads_to_rpm : Gain  Gain=30/pi
  MotPwrElecReq : Outport  VectorParamsAs1DForOutWhenUnconnected=off
  Eff2k : Outport  Port=2  VectorParamsAs1DForOutWhenUnconnected=off
  wires:
  Product3/1 -> Product4/1
  Switch2/1 -> Math Function/2
  Constant1/1 -> Switch2/1
  Constant2/1 -> Switch2/3
  Eff Map/1 -> Gain1/1
  Abs/1 -> Eff Map/1
  Gain1/1 -> Math Function/1
  Math Function/1 -> Eff2k/1, Product4/2
  Product4/1 -> MotPwrElecReq/1
  Abs1/1 -> Eff Map/2
  rads_to_rpm/1 -> Abs/1
  Product/1 -> Switch2/2
  MotSpd/1 -> Product3/1, Product/1, rads_to_rpm/1
  MotTrqCmd/1 -> Product3/2, Product/2, Abs1/1

== system CAVE_MachE_Simulink_250904_Test/Vehicle Under Test1/Vehicle/Powertrain Supervisory Controller /Engine Torque Command/Motor Torque Arbitration and Power Management/Power Management/Torque Limit ==
  MotTrq : Inport
  MotSpd : Inport  Port=2
  Gain : Gain  Gain=-1
  Max Motor Torque : LibPtSupervisoryCtrl/Powertrain Supervisory Controller /Engine Torque Command/Accel Pedal to Traction Wheel Torque Request/Max Motor Torque  SystemSampleTime=-1  VariantActivationTime=update diagram  AllowFlexibleInterface=on  Latency=0  AutoFrameSizeCalculation=off
  Saturation Dynamic : simulink/Discontinuities/Saturation Dynamic  OutMin=[]  OutMax=[]  OutDataTypeStr=Inherit: Same as second input  OutDataType=fixdt(1, 16)  OutScaling=2^-10  DoSatur=off
  MotTrqCmd : Outport  VectorParamsAs1DForOutWhenUnconnected=off
  wires:
  MotTrq/1 -> Saturation Dynamic/2
  Saturation Dynamic/1 -> MotTrqCmd/1
  Max Motor Torque/1 -> Gain/1, Saturation Dynamic/1
  Gain/1 -> Saturation Dynamic/3
  MotSpd/1 -> Max Motor Torque/1

== system CAVE_MachE_Simulink_250904_Test/Vehicle Under Test1/Vehicle/Rototest and ORNL Interface/Get Wheel Spd Cmd Based on Wheel Dynamics/Whl Dynamics & Format CM Powertrain Signal/Subsystem/WheelInertia ==
  In1 : Inport
  Divide : Product  Inputs=*/
  Switch : Switch  Criteria=u2 ~= 0  ZeroCross=off  SaturateOnIntegerOverflow=off  InputSameDT=off
  Zero : Constant
  Zero1 : Constant  Value=0.74063
  Out1 : Outport
  wires:
  Divide/1 -> Out1/1
  In1/1 -> Divide/1
  Zero/1 -> Switch/3
  Switch/1 -> Divide/2
  Zero1/1 -> Switch/2, Switch/1

== system CAVE_MachE_Simulink_250904_Test/Vehicle Under Test1/Vehicle/Rototest and ORNL Interface/Get Wheel Spd Cmd Based on Wheel Dynamics/Whl Dynamics & Format CM Powertrain Signal/Subsystem/WheelInertia1 ==
  In1 : Inport
  Divide : Product  Inputs=*/
  Switch : Switch  Criteria=u2 ~= 0  ZeroCross=off  SaturateOnIntegerOverflow=off  InputSameDT=off
  Zero : Constant
  Zero1 : Constant  Value=0.82
  axleTorq : Outport
  wires:
  Divide/1 -> axleTorq/1
  In1/1 -> Divide/1
  Zero/1 -> Switch/3
  Switch/1 -> Divide/2
  Zero1/1 -> Switch/2, Switch/1

== system CAVE_MachE_Simulink_250904_Test/Vehicle Under Test1/Vehicle/Rototest and ORNL Interface/Get Wheel Spd Cmd Based on Wheel Dynamics/Whl Dynamics & Format CM Powertrain Signal/Subsystem1/WheelInertia ==
  In1 : Inport
  Divide : Product  Inputs=*/
  Read CM Parameter : CarMaker4SL/Read CM Parameter  xfile=Vehicle  xkey=Wheel.fl.I  xnout=3  xdefaults=[]  xmuxed=off  xstime=Continuous
      settings: SourceProductName=CarMaker4SL
  Switch : Switch  Criteria=u2 ~= 0  ZeroCross=off  SaturateOnIntegerOverflow=off  InputSameDT=off
  Terminator : Terminator
  Terminator1 : Terminator
  Zero : Constant
  Out1 : Outport
  wires:
  Divide/1 -> Out1/1
  Read CM Parameter/1 -> Terminator/1
  Read CM Parameter/3 -> Terminator1/1
  In1/1 -> Divide/1
  Zero/1 -> Switch/3
  Switch/1 -> Divide/2
  Read CM Parameter/2 -> Switch/2, Switch/1

== system CAVE_MachE_Simulink_250904_Test/Vehicle Under Test1/Vehicle/Rototest and ORNL Interface/Get Wheel Spd Cmd Based on Wheel Dynamics/Whl Dynamics & Format CM Powertrain Signal/Subsystem2/WheelInertia ==
  In1 : Inport
  Divide : Product  Inputs=*/
  Switch : Switch  Criteria=u2 ~= 0  ZeroCross=off  SaturateOnIntegerOverflow=off  InputSameDT=off
  Zero : Constant
  Zero1 : Constant  Value=0.74063
  Out1 : Outport
  wires:
  Divide/1 -> Out1/1
  In1/1 -> Divide/1
  Zero/1 -> Switch/3
  Switch/1 -> Divide/2
  Zero1/1 -> Switch/2, Switch/1

== system CAVE_MachE_Simulink_250904_Test/Vehicle Under Test1/Vehicle/Rototest and ORNL Interface/Get Wheel Spd Cmd Based on Wheel Dynamics/Whl Dynamics & Format CM Powertrain Signal/Subsystem2/WheelInertia1 ==
  In1 : Inport
  Divide : Product  Inputs=*/
  Switch : Switch  Criteria=u2 ~= 0  ZeroCross=off  SaturateOnIntegerOverflow=off  InputSameDT=off
  Zero : Constant
  Zero1 : Constant  Value=0.82
  Out1 : Outport
  wires:
  Divide/1 -> Out1/1
  In1/1 -> Divide/1
  Zero/1 -> Switch/3
  Switch/1 -> Divide/2
  Zero1/1 -> Switch/2, Switch/1

== system CAVE_MachE_Simulink_250904_Test/Vehicle Under Test1/Vehicle/Rototest and ORNL Interface/Get Wheel Spd Cmd Based on Wheel Dynamics/Whl Dynamics & Format CM Powertrain Signal/Subsystem3/WheelInertia ==
  In1 : Inport
  Divide : Product  Inputs=*/
  Switch : Switch  Criteria=u2 ~= 0  ZeroCross=off  SaturateOnIntegerOverflow=off  InputSameDT=off
  Zero : Constant
  Zero1 : Constant  Value=0.74063
  Out1 : Outport
  wires:
  Divide/1 -> Out1/1
  In1/1 -> Divide/1
  Zero/1 -> Switch/3
  Switch/1 -> Divide/2
  Zero1/1 -> Switch/2, Switch/1

== system CAVE_MachE_Simulink_250904_Test/Vehicle Under Test1/Vehicle/Rototest and ORNL Interface/Get Wheel Spd Cmd Based on Wheel Dynamics/Whl Dynamics & Format CM Powertrain Signal/Subsystem3/WheelInertia1 ==
  In1 : Inport
  Divide : Product  Inputs=*/
  Switch : Switch  Criteria=u2 ~= 0  ZeroCross=off  SaturateOnIntegerOverflow=off  InputSameDT=off
  Zero : Constant
  Zero1 : Constant  Value=0.82
  axleTorq : Outport
  wires:
  Divide/1 -> axleTorq/1
  In1/1 -> Divide/1
  Zero/1 -> Switch/3
  Switch/1 -> Divide/2
  Zero1/1 -> Switch/2, Switch/1

== system CAVE_MachE_Simulink_250904_Test/Vehicle Under Test1/Vehicle/Rototest and ORNL Interface/Get Wheel Spd Cmd Based on Wheel Dynamics/Whl Dynamics & Format CM Powertrain Signal/Subsystem4/WheelInertia ==
  In1 : Inport
  Divide : Product  Inputs=*/
  Switch : Switch  Criteria=u2 ~= 0  ZeroCross=off  SaturateOnIntegerOverflow=off  InputSameDT=off
  Zero : Constant
  Zero1 : Constant  Value=0.74063
  Out1 : Outport
  wires:
  Divide/1 -> Out1/1
  In1/1 -> Divide/1
  Zero/1 -> Switch/3
  Switch/1 -> Divide/2
  Zero1/1 -> Switch/2, Switch/1

== system CAVE_MachE_Simulink_250904_Test/Vehicle Under Test1/Vehicle/Rototest and ORNL Interface/Get Wheel Spd Cmd Based on Wheel Dynamics/Whl Dynamics & Format CM Powertrain Signal/Subsystem4/WheelInertia1 ==
  In1 : Inport
  Divide : Product  Inputs=*/
  Switch : Switch  Criteria=u2 ~= 0  ZeroCross=off  SaturateOnIntegerOverflow=off  InputSameDT=off
  Zero : Constant
  Zero1 : Constant  Value=0.82
  axleTorq : Outport
  wires:
  Divide/1 -> axleTorq/1
  In1/1 -> Divide/1
  Zero/1 -> Switch/3
  Switch/1 -> Divide/2
  Zero1/1 -> Switch/2, Switch/1

== system CAVE_MachE_Simulink_250904_Test/Vehicle Under Test1/Vehicle/Rototest and ORNL Interface/Get Wheel Spd Cmd Based on Wheel Dynamics/Whl Dynamics & Format CM Powertrain Signal/Subsystem5/WheelInertia1 ==
  In1 : Inport
  Divide : Product  Inputs=*/
  Read CM Parameter : CarMaker4SL/Read CM Parameter  xfile=Vehicle  xkey=Wheel.fr.I  xnout=3  xdefaults=[]  xmuxed=off  xstime=Continuous
      settings: SourceProductName=CarMaker4SL
  Switch : Switch  Criteria=u2 ~= 0  ZeroCross=off  SaturateOnIntegerOverflow=off  InputSameDT=off
  Terminator : Terminator
  Terminator1 : Terminator
  Zero : Constant
  Out1 : Outport
  wires:
  Switch/1 -> Divide/2
  Zero/1 -> Switch/3
  Read CM Parameter/2 -> Switch/1, Switch/2
  In1/1 -> Divide/1
  Read CM Parameter/3 -> Terminator1/1
  Read CM Parameter/1 -> Terminator/1
  Divide/1 -> Out1/1

== system CAVE_MachE_Simulink_250904_Test/Vehicle Under Test1/Vehicle/Rototest and ORNL Interface/Get Wheel Spd Cmd Based on Wheel Dynamics/Whl Dynamics & Format CM Powertrain Signal/Subsystem6/WheelInertia2 ==
  In1 : Inport
  Divide : Product  Inputs=*/
  Read CM Parameter : CarMaker4SL/Read CM Parameter  xfile=Vehicle  xkey=Wheel.rl.I  xnout=3  xdefaults=[]  xmuxed=off  xstime=Continuous
      settings: SourceProductName=CarMaker4SL
  Switch : Switch  Criteria=u2 ~= 0  ZeroCross=off  SaturateOnIntegerOverflow=off  InputSameDT=off
  Terminator : Terminator
  Terminator1 : Terminator
  Zero : Constant
  Out1 : Outport
  wires:
  Divide/1 -> Out1/1
  Read CM Parameter/1 -> Terminator/1
  Read CM Parameter/3 -> Terminator1/1
  In1/1 -> Divide/1
  Read CM Parameter/2 -> Switch/2, Switch/1
  Zero/1 -> Switch/3
  Switch/1 -> Divide/2

== system CAVE_MachE_Simulink_250904_Test/Vehicle Under Test1/Vehicle/Rototest and ORNL Interface/Get Wheel Spd Cmd Based on Wheel Dynamics/Whl Dynamics & Format CM Powertrain Signal/Subsystem7/WheelInertia3 ==
  In1 : Inport
  Divide : Product  Inputs=*/
  Read CM Parameter : CarMaker4SL/Read CM Parameter  xfile=Vehicle  xkey=Wheel.rr.I  xnout=3  xdefaults=[]  xmuxed=off  xstime=Continuous
      settings: SourceProductName=CarMaker4SL
  Switch : Switch  Criteria=u2 ~= 0  ZeroCross=off  SaturateOnIntegerOverflow=off  InputSameDT=off
  Terminator : Terminator
  Terminator1 : Terminator
  Zero : Constant
  Out1 : Outport
  wires:
  Switch/1 -> Divide/2
  Zero/1 -> Switch/3
  Read CM Parameter/2 -> Switch/1, Switch/2
  In1/1 -> Divide/1
  Read CM Parameter/3 -> Terminator1/1
  Read CM Parameter/1 -> Terminator/1
  Divide/1 -> Out1/1
